simulink model "FirstStateflow"  (R2024a)
settings: Solver=VariableStepAuto  StartTime=0.0  StopTime=100.0  RelTol=1e-3
settings Model: Creator=pasqualederosa  LastModifiedBy=pasqualederosa

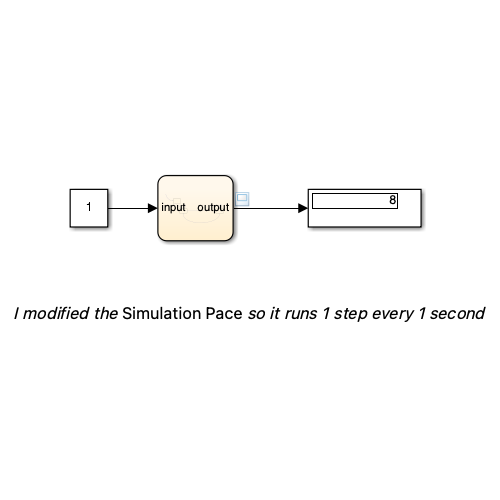
[thumbnail: Simulink's stored preview of the top-level diagram]
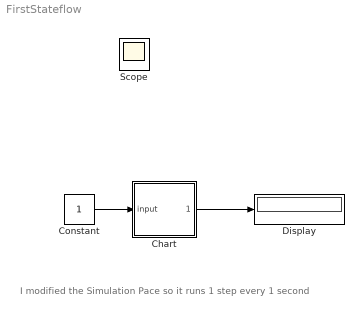
== system FirstStateflow ==
  note: I modified the Simulation Pace so it runs 1 step every 1 second
  Chart : Stateflow chart  TreatAsAtomicUnit=on
  Constant : Constant
  Display : Display
  Scope : Scope
  wires:
  Constant/1 -> Chart/1(input)
  Chart/1(output) -> Display/1

== stateflow chart FirstStateflow/Chart ==
  state State0
    x=0;
    output=x;
  state State1
    x = x + input;
    output=x;
  state State2
    x = x - 1
    output=x;
  (default) -> State0
  State0 -> State1
  State2 -> State2 [order 2] : [x>=5]
  State1 -> State1 [order 2] : [x<=10]
  State1 -> State2 [order 1] : [x>10]
  State2 -> State1 [order 1] : [x<5]
  data: x local; input input; output output
